simulink library "Library_Muscle_implementation_Ver_01"  (R2020a)
settings: Solver=VariableStepAuto  StartTime=0.0  StopTime=10.0  RelTol=1e-3
undefined symbols (not defined in the file or in its folder): Gait_trajectory_matrix, Param_Mus, X, Y, Z
libraries: sm_lib x8, $bdroot x3, nesl_utility x3, simulink x1, simulink_extras x1
settings Model: Creator=Tobi  LastModifiedBy=Tobi

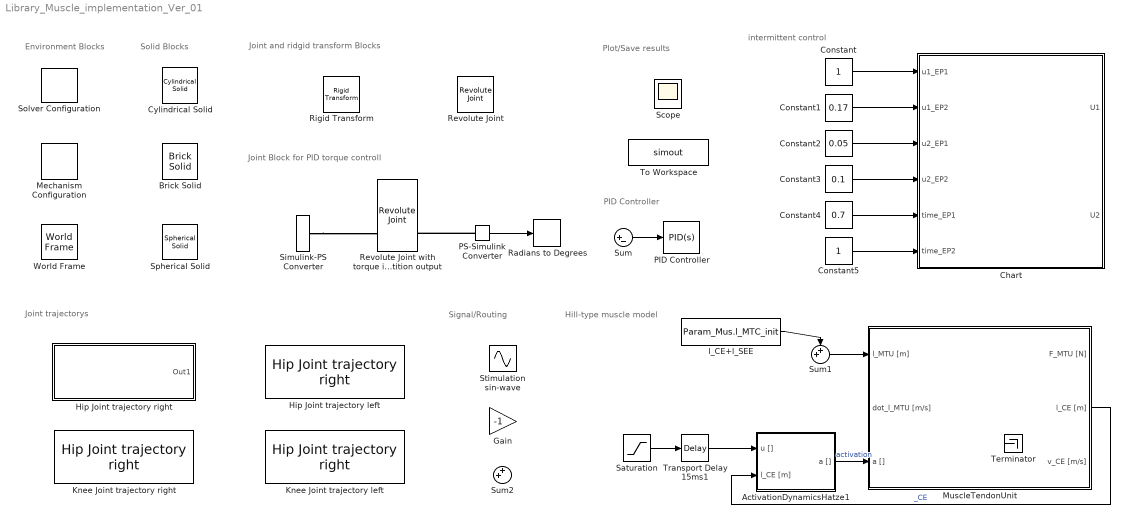
== system Library_Muscle_implementation_Ver_01 ==
  note: Signal/Routing
  note: intermittent control
  note: Joint trajectorys
  note: Plot/Save results
  note: Joint Block for PID torque controll
  note: Solid Blocks
  note: Joint and ridgid transform Blocks
  note: Environment Blocks
  note: PID Controller
  note: Hill-type muscle model
  ActivationDynamicsHatze1 : Subsystem  mask(Activation Dynamics){Act_Param=Param_Mus.ActDyn, Mus_Param=Param_Mus}
      mask prompts: Act_Param "Activation Parameter Struct"; Mus_Param "Muscle Parameter Struct"
      mask help:
      | This block solves the ODE linking neural muscle stimulation u(t) to muscle
      | activity a(t).
      mask Display: %text(.35,.3, 'Aktivierung')
  Brick Solid : sm_lib/Body Elements/Brick Solid  GraphicAmbientColor=[0.15 0.15 0.15 1.0]  BasedOnType=Density  BrickDimensions=[1 1 1]  BrickDimensionUnits=m  CenterOfMass=[0 0 0]  CenterOfMassUnits=m  GraphicDiffuseColor=[0.5 0.5 0.5]  Density=1000  DensityUnits=kg/m^3  DoExposeReferenceFrame=on  GraphicEmissiveColor=[0.0 0.0 0.0 1.0]  ExportEntireGeometry=off  SerializedFrames=<Frames/>  MarkerShape=Sphere  MarkerSize=10  GraphicType=FromGeometry  InertiaType=CalculateFromGeometry  Mass=1  MassUnits=kg  MomentsOfInertia=[1 1 1]  MomentsOfInertiaUnits=kg*m^2  GraphicOpacity=1.0  ProductsOfInertia=[0 0 0]  ProductsOfInertiaUnits=kg*m^2  GraphicShininess=75  GraphicSpecularColor=[0.5 0.5 0.5 1.0]  GraphicVisPropType=SimpleVisualProperties
  Chart : Stateflow chart  TreatAsAtomicUnit=on
  Constant : Constant
  Constant1 : Constant  Value=0.17
  Constant2 : Constant  Value=0.05
  Constant3 : Constant  Value=0.1
  Constant4 : Constant  Value=0.7
  Constant5 : Constant
  Cylindrical Solid : sm_lib/Body Elements/Cylindrical Solid  GraphicAmbientColor=[0.15 0.15 0.15 1.0]  BasedOnType=Density  CenterOfMass=[0 0 0]  CenterOfMassUnits=m  GraphicDiffuseColor=[0.5 0.5 0.5]  CylinderLength=1  CylinderLengthUnits=m  CylinderRadius=1  CylinderRadiusUnits=m  Density=1000  DensityUnits=kg/m^3  DoExposeReferenceFrame=on  GraphicEmissiveColor=[0.0 0.0 0.0 1.0]  ExportEntireGeometry=off  SerializedFrames=<Frames/>  MarkerShape=Sphere  MarkerSize=10  GraphicType=FromGeometry  InertiaType=CalculateFromGeometry  Mass=1  MassUnits=kg  MomentsOfInertia=[1 1 1]  MomentsOfInertiaUnits=kg*m^2  GraphicOpacity=1.0  ProductsOfInertia=[0 0 0]  ProductsOfInertiaUnits=kg*m^2  GraphicShininess=75  GraphicSpecularColor=[0.5 0.5 0.5 1.0]  GraphicVisPropType=SimpleVisualProperties
  Gain : Gain  Gain=-1
  Hip Joint trajectory left : $bdroot/Hip Joint trajectory right   SystemSampleTime=-1  Latency=0  AutoFrameSizeCalculation=off
      link override n-D Lookup Table: Table=Gait_trajectory_matrix(:,2)
  "Hip Joint trajectory right " : Subsystem
  Knee Joint trajectory left : $bdroot/Hip Joint trajectory right   SystemSampleTime=-1  Latency=0  AutoFrameSizeCalculation=off
      link override n-D Lookup Table: Table=Gait_trajectory_matrix(:,4)
  Knee Joint trajectory right : $bdroot/Hip Joint trajectory right   SystemSampleTime=-1  Latency=0  AutoFrameSizeCalculation=off
      link override n-D Lookup Table: Table=Gait_trajectory_matrix(:,5)
  Mechanism Configuration : sm_lib/Utilities/Mechanism Configuration  UniformGravity=Constant  GravityVector=[0 0 -9.80665]  GravityUnits=m/s^2  LinearizationDelta=0.001
  MuscleTendonUnit : Subsystem  mask(Muscle Tendon Complex Model){Mus_Param=Param_Mus}
      mask prompts: Mus_Param "Muscle parameter struct"
      mask help: This block returns the muscle tendon complex (MTC) force based on muscle length l_MTC, contraction velocity dot_l_MTC, and activity q
      mask Help:
      | Copyright (c) 2013, D. Haeufle, M. Guenther, A. Bayer, and S. Schmitt
      | All rights reserved.
      | 
      | Redistribution and use in source and binary forms, with or without modification, are permitted provided that the following conditions are met:
      | 
      |     Redistributions of source code must retain the above copyright notice, this list of conditions and the following disclaimer.
      |     Redistributions in binary form must reproduce the above copyright notice, this list of conditions and the following disclaimer in the documentation and/or other materials provided with the distribution.
      |     Neither the name of the <ORGANIZATION> nor the names of its contributors may be used to endorse or promote products derived from this software without specific prior written permission.
      | 
      | THIS SOFTWARE IS PROVIDED BY THE COPYRIGHT HOLDERS AND CONTRIBUTORS "AS IS" AND ANY EXPRESS OR IMPLIED WARRANTIES, INCLUDING, BUT NOT LIMITED TO, THE IMPLIED WARRANTIES OF MERCHANTABILITY AND FITNESS FOR A PARTICULAR PURPOSE ARE DISCLAIMED. IN NO EVENT SHALL THE COPYRIGHT HOLDER OR CONTRIBUTORS BE LIABLE FOR ANY DIRECT, INDIRECT, INCIDENTAL, SPECIAL, EXEMPLARY, OR CONSEQUENTIAL DAMAGES (INCLUDING, BUT NOT LIMITED TO, PROCUREMENT OF SUBSTITUTE GOODS OR SERVICES; LOSS OF USE, DATA, OR PROFITS; OR BUSINESS INTERRUPTION) HOWEVER CAUSED AND ON ANY THEORY OF LIABILITY, WHETHER IN CONTRACT, STRICT LIABILITY, OR TORT (INCLUDING NEGLIGENCE OR OTHERWISE) ARISING IN ANY WAY OUT OF THE USE OF THIS SOFTWARE, EVEN IF ADVISED OF THE POSSIBILITY OF SUCH DAMAGE.
      mask Display: patch([4 4 4 4 3.5 3 2.6 2.2 2 2.2 2.6 3 3.5 4 4 4 4 7 7 7 7 7.5 8 8.4 8.8 9 8.8 8.4 8 7.5 7 7 7 7 4]/20+0.2, [0 2:17 17:-1:2 0 0]/17,[1 0 0])
  PID Controller : simulink/Continuous/PID Controller  Controller=PID  Form=Parallel  TimeDomain=Continuous-time  UseExternalTs=off  SampleTime=-1  IntegratorMethod=Forward Euler  FilterMethod=Forward Euler  ControllerParametersSource=internal  P=1  I=1  D=0  UseFilter=on  N=100  TunerSelectOption=Transfer Function Based (PID Tuner App)  InitialConditionSource=internal  InitialConditionForIntegrator=0  InitialConditionForFilter=0  DifferentiatorICPrevScaledInput=0  ExternalReset=none  TrackingMode=off  Kt=1  LimitOutput=off  UpperSaturationLimit=inf  LowerSaturationLimit=-inf  LinearizeAsGain=on  AntiWindupMode=none  Kb=1  POutMin=[]  POutMax=[]  IOutMin=[]  IOutMax=[]  DOutMin=[]  DOutMax=[]  NOutMin=[]  NOutMax=[]  SumOutMin=[]  SumOutMax=[]  SaturationOutMin=[]  SaturationOutMax=[]  PParamMin=[]  PParamMax=[]  IParamMin=[]  IParamMax=[]  DParamMin=[]  DParamMax=[]  NParamMin=[]  NParamMax=[]  KbParamMin=[]  KbParamMax=[]  KtParamMin=[]  KtParamMax=[]  KbOutMin=[]  KbOutMax=[]  KtOutMin=[]  KtOutMax=[]  IntegratorOutMin=[]  IntegratorOutMax=[]  FilterOutMin=[]  FilterOutMax=[]  SumI1OutMin=[]  SumI1OutMax=[]  SumI2OutMin=[]  SumI2OutMax=[]  SumI3OutMin=[]  SumI3OutMax=[]  SumI4OutMin=[]  SumI4OutMax=[]  SumDOutMin=[]  SumDOutMax=[]  DifferentiatorOutMin=[]  DifferentiatorOutMax=[]  FilterDiffOutCoefMin=[]  FilterDiffOutCoefMax=[]  ReciprocalOutMin=[]  ReciprocalOutMax=[]  SumDenOutMin=[]  SumDenOutMax=[]  SumNumOutMin=[]  SumNumOutMax=[]  DivideOutMin=[]  DivideOutMax=[]  UdiffTsProdOutMin=[]  UdiffTsProdOutMax=[]  NTsProdOutMin=[]  NTsProdOutMax=[]  UintegralTsProdOutMin=[]  UintegralTsProdOutMax=[]  UngainTsProdOutMin=[]  UngainTsProdOutMax=[]  IntegratorContinuousStateAttributes=''  IntegratorStateMustResolveToSignalObject=off  IntegratorRTWStateStorageClass=Auto  FilterContinuousStateAttributes=''  FilterStateMustResolveToSignalObject=off  FilterRTWStateStorageClass=Auto  ParallelPVariant=InternalParameters  IdealPVariant=Disabled  IVariant=InternalParameters  DVariant=InternalParameters  IntegratorVariant=Continuous  SatVariant=Disabled  AWVariant=Passthrough  PCopyVariant=Disabled  TRVariant=Disabled  FdbkBlocksVariant=Forward  IdealPFdbkVariant=Disabled  SatFdbkVariant=Disabled  DerivativeFilterVariant=ContFilter  NVariant=InternalParameters  NCopyVariant=Disabled  FilterICVariant=InternalICsFilter  IntegratorICVariant=InternalICs  ExternalResetVariant=Disabled  TRSumVariant=Passthrough  SumFdbkVariant=Disabled  SumVariant=Sum_PID  TsampFilterVariant=InternalTs  TsampNgainVariant=Passthrough  TsampIntegralVariant=Passthrough
  PS-Simulink Converter : nesl_utility/PS-Simulink Converter  PhysicalDomain=network_engine_domain  SubClassName=ps_output  LeftPortType=input  RightPortType=output  PseudoPeriodic=off  Frequencies=[]  Unit=1  AffineConversion=off
  Radians to Degrees : simulink_extras/Transformations/Radians to Degrees
  Revolute Joint : sm_lib/Joints/Revolute Joint  JointMode=Normal  SenseConstraintForce=off  SenseConstraintForceX=off  SenseConstraintForceY=off  SenseConstraintForceZ=off  SenseConstraintTorque=off  SenseConstraintTorqueX=off  SenseConstraintTorqueY=off  SenseConstraintTorqueZ=off  SenseTotalForce=off  SenseTotalForceX=off  SenseTotalForceY=off  SenseTotalForceZ=off  SenseTotalTorque=off  SenseTotalTorqueX=off  SenseTotalTorqueY=off  SenseTotalTorqueZ=off  CompositeWrenchDir=FollowerOnBase  CompositeWrenchFrame=BaseFrame  EquilibriumPosition=0  EquilibriumPositionUnits=deg  SpringStiffness=0  SpringStiffnessUnits=N*m/deg  DampingCoefficient=0  DampingCoefficientUnits=N*m/(deg/s)  TorqueActuationMode=NoTorque  MotionActuationMode=ComputedMotion  SensePosition=off  SenseVelocity=off  SenseAcceleration=off  SenseTorqueForce=off  SenseLowerLimitTorqueForce=off  SenseUpperLimitTorqueForce=off  LowerLimitSpecify=off  LowerLimitBound=-90  LowerLimitBoundUnits=deg  LowerLimitStiffness=1e4  LowerLimitStiffnessUnits=N*m/deg  LowerLimitDamping=10  LowerLimitDampingUnits=N*m/(deg/s)  LowerLimitTransitionRegionWidth=0.1  LowerLimitTransitionRegionWidthUnits=deg  UpperLimitSpecify=off  UpperLimitBound=90  UpperLimitBoundUnits=deg  UpperLimitStiffness=1e4  UpperLimitStiffnessUnits=N*m/deg  UpperLimitDamping=10  UpperLimitDampingUnits=N*m/(deg/s)  UpperLimitTransitionRegionWidth=0.1  UpperLimitTransitionRegionWidthUnits=deg  PositionTargetSpecify=off  PositionTargetPriority=High  PositionTargetValue=0  PositionTargetValueUnits=deg  VelocityTargetSpecify=off  VelocityTargetPriority=High  VelocityTargetValue=0  VelocityTargetValueUnits=deg/s
  "Revolute Joint with torque input and postition output " : sm_lib/Joints/Revolute Joint  JointMode=Normal  SenseConstraintForce=off  SenseConstraintForceX=off  SenseConstraintForceY=off  SenseConstraintForceZ=off  SenseConstraintTorque=off  SenseConstraintTorqueX=off  SenseConstraintTorqueY=off  SenseConstraintTorqueZ=off  SenseTotalForce=off  SenseTotalForceX=off  SenseTotalForceY=off  SenseTotalForceZ=off  SenseTotalTorque=off  SenseTotalTorqueX=off  SenseTotalTorqueY=off  SenseTotalTorqueZ=off  CompositeWrenchDir=FollowerOnBase  CompositeWrenchFrame=BaseFrame  EquilibriumPosition=0  EquilibriumPositionUnits=deg  SpringStiffness=0  SpringStiffnessUnits=N*m/deg  DampingCoefficient=0  DampingCoefficientUnits=N*m/(deg/s)  TorqueActuationMode=InputTorque  MotionActuationMode=ComputedMotion  SensePosition=on  SenseVelocity=off  SenseAcceleration=off  SenseTorqueForce=off  SenseLowerLimitTorqueForce=off  SenseUpperLimitTorqueForce=off  LowerLimitSpecify=off  LowerLimitBound=-90  LowerLimitBoundUnits=deg  LowerLimitStiffness=1e4  LowerLimitStiffnessUnits=N*m/deg  LowerLimitDamping=10  LowerLimitDampingUnits=N*m/(deg/s)  LowerLimitTransitionRegionWidth=0.1  LowerLimitTransitionRegionWidthUnits=deg  UpperLimitSpecify=off  UpperLimitBound=90  UpperLimitBoundUnits=deg  UpperLimitStiffness=1e4  UpperLimitStiffnessUnits=N*m/deg  UpperLimitDamping=10  UpperLimitDampingUnits=N*m/(deg/s)  UpperLimitTransitionRegionWidth=0.1  UpperLimitTransitionRegionWidthUnits=deg  PositionTargetSpecify=off  PositionTargetPriority=High  PositionTargetValue=0  PositionTargetValueUnits=deg  VelocityTargetSpecify=off  VelocityTargetPriority=High  VelocityTargetValue=0  VelocityTargetValueUnits=deg/s
  Rigid Transform : sm_lib/Frames and Transforms/Rigid Transform  TranslationMethod=Cartesian  TranslationStandardOffset=0  TranslationLengthUnit=m  TranslationStandardAxis=+Z  TranslationCartesianOffset=[0 0 0]  TranslationROffset=0  TranslationROffsetUnits=m  TranslationZOffset=0  TranslationZOffsetUnits=m  TranslationThetaOffset=0  TranslationThetaOffsetUnits=deg  RotationMethod=StandardAxis  RotationAngleUnits=deg  RotationStandardAxis=+X  RotationAngle=0.0  RotationArbitraryAxis=[0 0 1]  FollAlignAxisA=+X  BaseAlignAxisA=+Y  FollAlignAxisB=+Y  BaseAlignAxisB=+Z  RotationSequenceAxes=FollowerAxes  RotationSequence=XYX  RotationSequenceAngles=[0 0 0]  RotationSequenceAnglesUnits=deg  RotationMatrix=[1 0 0; 0 1 0; 0 0 1]
  Saturation : Saturate  UpperLimit=1  LowerLimit=0.001
  Scope : Scope
  Simulink-PS Converter : nesl_utility/Simulink-PS Converter  PhysicalDomain=network_engine_domain  SubClassName=ps_input  LeftPortType=input  RightPortType=output  PseudoPeriodic=off  Frequencies=[]  NoiseDistribution=none  NoiseParameters=[]  Unit=1  AffineConversion=off  FilteringAndDerivatives=zero  SimscapeFilterOrder=2  InputFilterTimeConstant=0.001  UdotUserProvided=0
  Solver Configuration : nesl_utility/Solver Configuration  PhysicalDomain=network_engine_domain  SubClassName=solver  LeftPortType=input  RightPortType=generic  Tones=[]  Harmonics=[]  SimulateNoise=off  Profile=off  UseLocalSampling=off  EnableSwitchedLinearOptims=on  FrequencyDomain=off  UseCCode=off  RelTol=0.001  AbsTol=1e-06  MinStep=1e-09  ToWorkspace=off  RevertToSquareIcSolve=off  NumHomotopyIterations=100  PhasorMode=off  PhasorModeNumHarmonics=1  DoDC=off  ResidualTolerance=1e-09  UseLocalSolver=off  LocalSolverChoice=NE_BACKWARD_EULER_ADVANCER  LocalSolverSampleTime=0.001  DoFixedCost=off  MaxNonlinIter=3  MaxModeIter=2  LinearAlgebra=auto  EquationFormulation=NE_TIME_EF  DelaysMemoryBudget=1024  AutomaticFiltering=on  FilteringTimeConstant=0.001  PartitionStorageMethod=AS_NEEDED  PartitionMemoryBudget=1024  PartitionMethod=ROBUST
  Spherical Solid : sm_lib/Body Elements/Spherical Solid  GraphicAmbientColor=[0.15 0.15 0.15 1.0]  BasedOnType=Density  CenterOfMass=[0 0 0]  CenterOfMassUnits=m  GraphicDiffuseColor=[0.0 0.0 0.0]  Density=1000  DensityUnits=kg/m^3  DoExposeReferenceFrame=on  GraphicEmissiveColor=[0.0 0.0 0.0 1.0]  ExportEntireGeometry=off  SerializedExposedGeometries=<ExposedGeometries/>  SerializedFrames=<Frames/>  MarkerShape=Sphere  MarkerSize=10  GraphicType=FromGeometry  InertiaType=PointMass  Mass=0  MassUnits=kg  MomentsOfInertia=[1 1 1]  MomentsOfInertiaUnits=kg*m^2  GraphicOpacity=1.0  ProductsOfInertia=[0 0 0]  ProductsOfInertiaUnits=kg*m^2  GraphicShininess=75  GraphicSpecularColor=[0.5 0.5 0.5 1.0]  SphereRadius=Joint_radius  SphereRadiusUnits=m  GraphicVisPropType=SimpleVisualProperties
  Stimulation sin-wave : Sin  Amplitude=0.25  Bias=0.45  Frequency=3  Phase=-pi/2  SampleTime=0
  Sum : Sum  Inputs=|+-
  Sum1 : Sum  Inputs=++|
  Sum2 : Sum  Inputs=++|
  Terminator : Terminator
  To Workspace : ToWorkspace  VariableName=simout  SaveFormat=Structure With Time  SampleTime=-1
  Transport Delay 15ms1 : TransportDelay  DelayTime=0.015  InitialOutput=Param_Mus.ActDyn.u_init
  World Frame : sm_lib/Frames and Transforms/World Frame
  l_CE+l_SEE : Constant  Value=Param_Mus.l_MTC_init
  wires:
  PS-Simulink Converter/1 -> Radians to Degrees/1
  Sum/1 -> PID Controller/1
  l_CE+l_SEE/1 -> Sum1/1
  MuscleTendonUnit/2(l_CE [m]) -> ActivationDynamicsHatze1/2(l_CE [m])  "_CE"
  Transport Delay 15ms1/1 -> ActivationDynamicsHatze1/1(u [])
  ActivationDynamicsHatze1/1(a []) -> MuscleTendonUnit/3(a [])  "activation"
  ? -> Terminator/1  "v_CE"
  Sum1/1 -> MuscleTendonUnit/1(l_MTU [m])
  Constant2/1 -> Chart/3(u2_EP1)
  Constant3/1 -> Chart/4(u2_EP2)
  Constant/1 -> Chart/1(u1_EP1)
  Constant1/1 -> Chart/2(u1_EP2)
  Constant4/1 -> Chart/5(time_EP1)
  Constant5/1 -> Chart/6(time_EP2)
  Saturation/1 -> Transport Delay 15ms1/1
  connections:
  PS-Simulink Converter/LConn1 -- "Revolute Joint with torque input and postition output "/RConn2
  Simulink-PS Converter/RConn1 -- "Revolute Joint with torque input and postition output "/LConn2

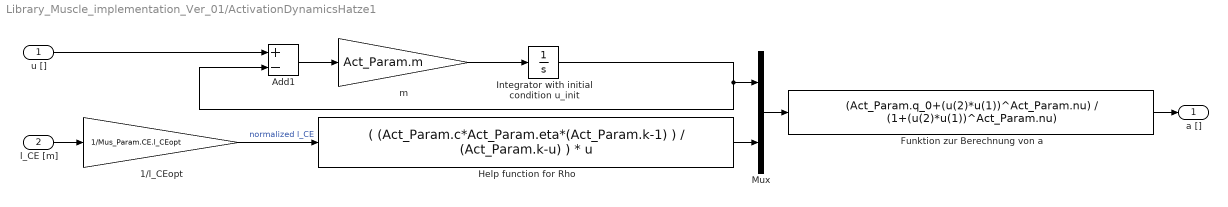
== system Library_Muscle_implementation_Ver_01/ActivationDynamicsHatze1 ==
  u [] : Inport
  l_CE [m] : Inport  Port=2
  1/l_CEopt : Gain  Gain=1/Mus_Param.CE.l_CEopt
  Add1 : Sum  Inputs=+-
  Funktion zur Berechnung von a : Fcn  Expr=(Act_Param.q_0+(u(2)*u(1))^Act_Param.nu) / (1+(u(2)*u(1))^Act_Param.nu)
  Help function for Rho : Fcn  Expr=( (Act_Param.c*Act_Param.eta*(Act_Param.k-1) ) / (Act_Param.k-u) ) * u
  Integrator with initial condition u_init : Integrator  InitialCondition=Act_Param.u_init
  Mux : Mux  Inputs=2
  m : Gain  Gain=Act_Param.m
  a [] : Outport  VectorParamsAs1DForOutWhenUnconnected=off
  wires:
  Add1/1 -> m/1
  m/1 -> Integrator with initial condition u_init/1
  Integrator with initial condition u_init/1 -> Add1/2, Mux/1
  Help function for Rho/1 -> Mux/2
  Mux/1 -> Funktion zur Berechnung von a/1
  l_CE [m]/1 -> 1/l_CEopt/1
  Funktion zur Berechnung von a/1 -> a []/1
  u []/1 -> Add1/1
  1/l_CEopt/1 -> Help function for Rho/1  "normalized l_CE"

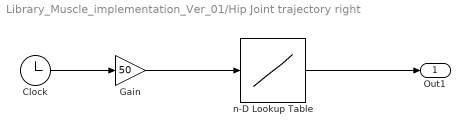
== system Library_Muscle_implementation_Ver_01/Hip Joint trajectory right  ==
  Clock : Clock
  Gain : Gain  Gain=50
  n-D Lookup Table : Lookup_n-D  NumberOfTableDimensions=1  BreakpointsSpecification=Even spacing  BreakpointsForDimension3=[5, 7]  Table=Gait_trajectory_matrix(:,3)  InternalRulePriority=Speed  RndMeth=Simplest  InputSameDT=on
  Out1 : Outport
  wires:
  n-D Lookup Table/1 -> Out1/1
  Clock/1 -> Gain/1
  Gain/1 -> n-D Lookup Table/1

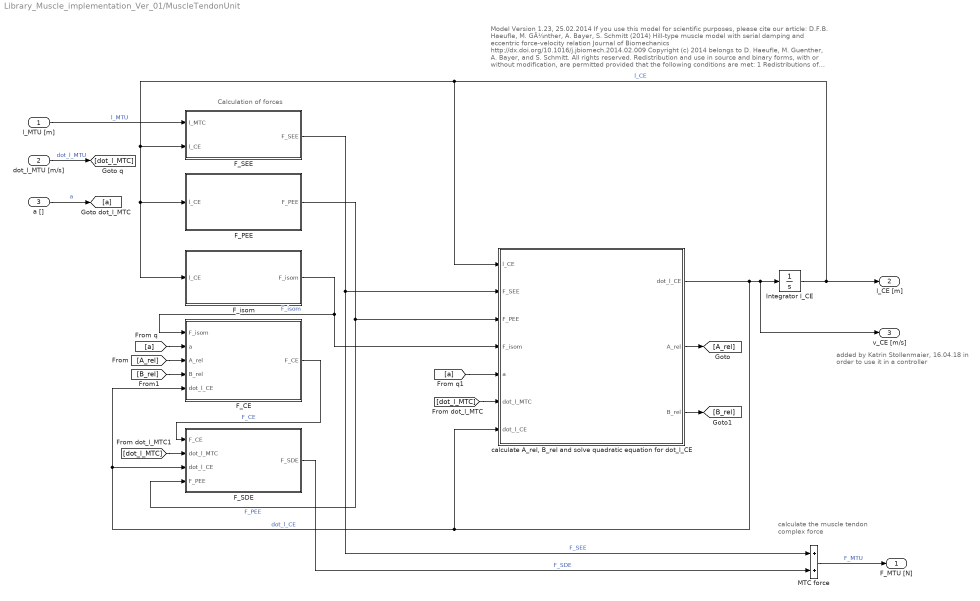
== system Library_Muscle_implementation_Ver_01/MuscleTendonUnit ==
  note: added by Katrin Stollenmaier,
      | 16.04.18 in order to use it in a controller
  note: Calculation of forces
  note: calculate the
      | muscle tendon complex
      | force
  note: Model Version 1.23, 25.02.2014
      |
      | If you use this model for scientific purposes, please cite our article:
      | D.F.B. Haeufle, M. GÃ¼nther, A. Bayer, S. Schmitt (2014)
      | Hill-type muscle model with serial damping and eccentric force-velocity relation
      | Journal of Biomechanics http://dx.doi.org/10.1016/j.jbiomech.2014.02.009
      |
      |
      | Copyright (c) 2014 belongs to D. Haeufle, M. Guenther, A. Bayer, and S. Schmitt. All rights reserved.
      | Redistribution and use in source and binary forms, with or without modification, are permitted provided that the following conditions are met:
      |
      |  1 Redistributions of source code must retain the above copyright notice,
      |    this list of conditions and the following disclaimer.
      |  2 Redistributions in binary form must reproduce the above copyright
      |    notice, this list of conditions and the following disclaimer in the
      |    documentation and/or other materials provided with the distribution.
      |  3 Neither the name of the owner nor the names of its contributors may be
      |    used to endorse or promote products derived from this software without
      |    specific prior written permission.
      |
      | THIS SOFTWARE IS PROVIDED BY THE COPYRIGHT HOLDERS AND CONTRIBUTORS "AS IS"
      | AND ANY EXPRESS OR IMPLIED WARRANTIES, INCLUDING, BUT NOT LIMITED TO, THE IMPLIED WARRANTIES OF
      | MERCHANTABILITY AND FITNESS FOR A PARTICULAR PURPOSE ARE DISCLAIMED.
      |  IN NO EVENT SHALL THE COPYRIGHT HOLDER BE LIABLE FOR ANY DIRECT, INDIRECT,
      | INCIDENTAL, SPECIAL, EXEMPLARY, OR CONSEQUENTIAL DAMAGES (INCLUDING, BUT
      | NOT LIMITED TO, PROCUREMENT OF SUBSTITUTE GOODS OR SERVICES; LOSS
      | OF USE, DATA, OR PROFITS; OR BUSINESS INTERRUPTION) HOWEVER CAUSED AND ON ANY
      | THEORY OF LIABILITY, WHETHER IN CONTRACT, STRICT LIABILITY, OR TORT (INCLUDING
      | NEGLIGENCE OR OTHERWISE) ARISING IN ANY WAY OUT OF THE USE OF THIS SOFTWARE,
      | EVEN IF ADVISED OF THE POSSIBILITY OF SUCH DAMAGE.
  l_MTU [m] : Inport
  dot_l_MTU [m/s] : Inport  Port=2
  a [] : Inport  Port=3
  F_CE : Subsystem
  F_PEE : Subsystem
  F_SDE : Subsystem
  F_SEE : Subsystem
  F_isom : Subsystem
  Integrator l_CE : Integrator  InitialCondition=Mus_Param.CE.l_CE_init
  MTC force : Sum
  "calculate A_rel, B_rel and solve quadratic equation for dot_l_CE" : Subsystem
  F_MTU [N] : Outport  VectorParamsAs1DForOutWhenUnconnected=off
  l_CE [m] : Outport  Port=2  VectorParamsAs1DForOutWhenUnconnected=off
  "v_CE [m/s] " : Outport  Port=3  VectorParamsAs1DForOutWhenUnconnected=off
  wires:
  F_isom/1(F_isom) -> "calculate A_rel, B_rel and solve quadratic equation for dot_l_CE"/4(F_isom), F_CE/1(F_isom)  "F_isom"
  F_PEE/1(F_PEE) -> F_SDE/4(F_PEE), "calculate A_rel, B_rel and solve quadratic equation for dot_l_CE"/3(F_PEE)  "F_PEE"
  F_SEE/1(F_SEE) -> MTC force/1, "calculate A_rel, B_rel and solve quadratic equation for dot_l_CE"/2(F_SEE)  "F_SEE"
  Integrator l_CE/1 -> l_CE [m]/1, "calculate A_rel, B_rel and solve quadratic equation for dot_l_CE"/1(l_CE), F_SEE/2(l_CE), F_isom/1(l_CE), F_PEE/1(l_CE)  "l_CE"
  F_CE/1(F_CE) -> F_SDE/1(F_CE)  "F_CE"
  F_SDE/1(F_SDE) -> MTC force/2  "F_SDE"
  MTC force/1 -> F_MTU [N]/1  "F_MTU"
  l_MTU [m]/1 -> F_SEE/1(l_MTC)  "l_MTU"
  "calculate A_rel, B_rel and solve quadratic equation for dot_l_CE"/1("dot_l_CE ") -> "calculate A_rel, B_rel and solve quadratic equation for dot_l_CE"/7(dot_l_CE), F_CE/5(dot_l_CE), F_SDE/3(dot_l_CE), "v_CE [m/s] "/1, Integrator l_CE/1  "dot_l_CE"
  [a] -> F_CE/2(a)
  [a] -> "calculate A_rel, B_rel and solve quadratic equation for dot_l_CE"/5("a ")
  [dot_l_MTC] -> "calculate A_rel, B_rel and solve quadratic equation for dot_l_CE"/6(dot_l_MTC)
  [dot_l_MTC] -> F_SDE/2(dot_l_MTC)
  "calculate A_rel, B_rel and solve quadratic equation for dot_l_CE"/2(A_rel) -> [A_rel]
  "calculate A_rel, B_rel and solve quadratic equation for dot_l_CE"/3(B_rel) -> [B_rel]
  [A_rel] -> F_CE/3(A_rel)
  [B_rel] -> F_CE/4(B_rel)
  dot_l_MTU [m/s]/1 -> [dot_l_MTC]  "dot_l_MTU"
  a []/1 -> [a]  "a"

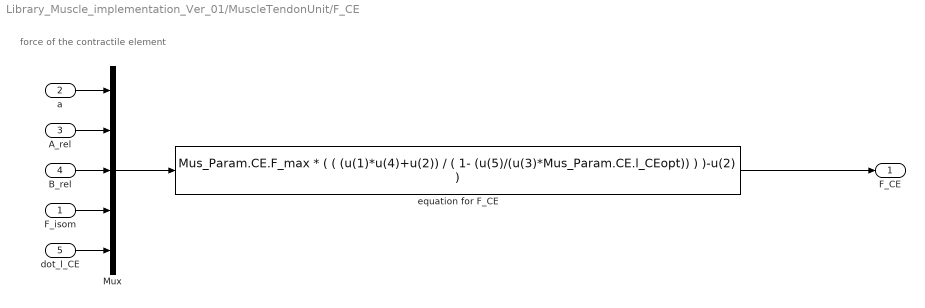
== system Library_Muscle_implementation_Ver_01/MuscleTendonUnit/F_CE ==
  note: force of the contractile element
  F_isom : Inport
  a : Inport  Port=2
  A_rel : Inport  Port=3
  B_rel : Inport  Port=4
  dot_l_CE : Inport  Port=5
  Mux : Mux  Inputs=5
  equation for F_CE : Fcn  Expr="Mus_Param.CE.F_max * (  ( (u(1)*u(4)+u(2)) / ( 1- (u(5)/(u(3)*Mus_Param.CE.l_CEopt)) ) )-u(2) )"
  F_CE : Outport  VectorParamsAs1DForOutWhenUnconnected=off
  wires:
  Mux/1 -> equation for F_CE/1
  a/1 -> Mux/1
  A_rel/1 -> Mux/2
  B_rel/1 -> Mux/3
  F_isom/1 -> Mux/4
  dot_l_CE/1 -> Mux/5
  equation for F_CE/1 -> F_CE/1

== system Library_Muscle_implementation_Ver_01/MuscleTendonUnit/F_PEE ==
  note: Parallel elastic element force
      |
      | is only calculated if l_CE>PEE slack length
      | to avoid complex numbers with
      | non-integer exponents
  l_CE : Inport
  "F_PEE " : Subsystem
  l_PEE > slack length? : Fcn  Expr=(u>=Mus_Param.PEE.l_PEE0)
  F_PEE : Outport  VectorParamsAs1DForOutWhenUnconnected=off
  wires:
  l_CE/1 -> l_PEE > slack length?/1, "F_PEE "/1(l_PEE)
  "F_PEE "/1(Out1) -> F_PEE/1
  l_PEE > slack length?/1 -> "F_PEE "/Enable

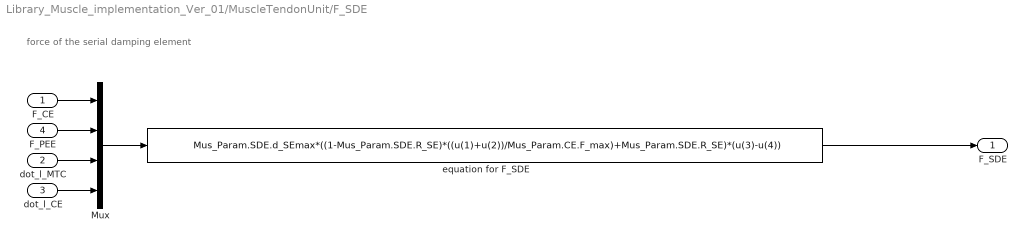
== system Library_Muscle_implementation_Ver_01/MuscleTendonUnit/F_SDE ==
  note: force of the serial damping element
  F_CE : Inport
  dot_l_MTC : Inport  Port=2
  dot_l_CE : Inport  Port=3
  F_PEE : Inport  Port=4
  Mux : Mux
  equation for F_SDE : Fcn  Expr=Mus_Param.SDE.d_SEmax*((1-Mus_Param.SDE.R_SE)*((u(1)+u(2))/Mus_Param.CE.F_max)+Mus_Param.SDE.R_SE)*(u(3)-u(4))
  F_SDE : Outport  VectorParamsAs1DForOutWhenUnconnected=off
  wires:
  Mux/1 -> equation for F_SDE/1
  F_PEE/1 -> Mux/2
  F_CE/1 -> Mux/1
  equation for F_SDE/1 -> F_SDE/1
  dot_l_MTC/1 -> Mux/3
  dot_l_CE/1 -> Mux/4

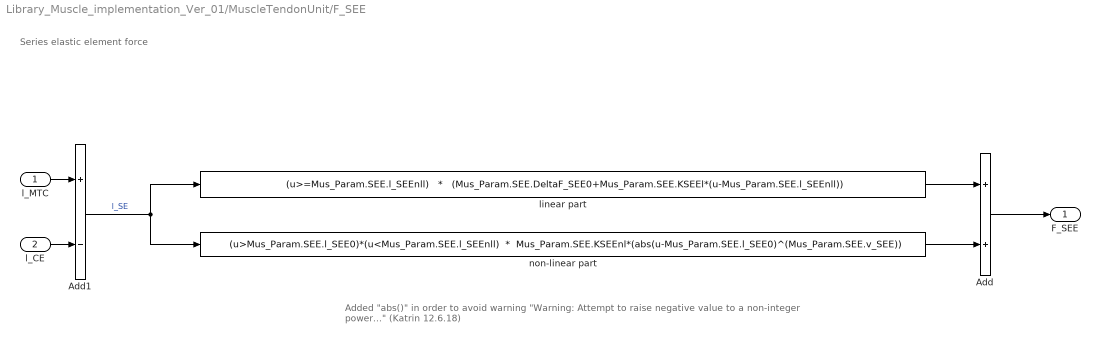
== system Library_Muscle_implementation_Ver_01/MuscleTendonUnit/F_SEE ==
  note: Added "abs()" in order to avoid warning "Warning: Attempt to raise negative value to a non-integer power..."
      | (Katrin 12.6.18)
  note: Series elastic element force
  l_MTC : Inport
  l_CE : Inport  Port=2
  Add : Sum
  Add1 : Sum  Inputs=+-
  linear part : Fcn  Expr="(u>=Mus_Param.SEE.l_SEEnll)   *   (Mus_Param.SEE.DeltaF_SEE0+Mus_Param.SEE.KSEEl*(u-Mus_Param.SEE.l_SEEnll))"
  non-linear part : Fcn  Expr="(u>Mus_Param.SEE.l_SEE0)*(u<Mus_Param.SEE.l_SEEnll)  *  Mus_Param.SEE.KSEEnl*(abs(u-Mus_Param.SEE.l_SEE0)^(Mus_Param.SEE.v_SEE))"
  F_SEE : Outport  VectorParamsAs1DForOutWhenUnconnected=off
  wires:
  linear part/1 -> Add/1
  Add1/1 -> linear part/1, non-linear part/1  "l_SE"
  l_MTC/1 -> Add1/1
  Add/1 -> F_SEE/1
  l_CE/1 -> Add1/2
  non-linear part/1 -> Add/2

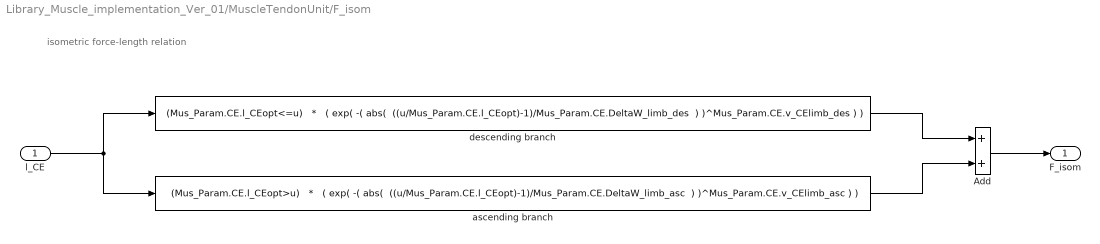
== system Library_Muscle_implementation_Ver_01/MuscleTendonUnit/F_isom ==
  note: isometric force-length relation
  l_CE : Inport
  Add : Sum
  ascending branch : Fcn  Expr="(Mus_Param.CE.l_CEopt>u)   *   ( exp( -( abs(  ((u/Mus_Param.CE.l_CEopt)-1)/Mus_Param.CE.DeltaW_limb_asc  ) )^Mus_Param.CE.v_CElimb_asc ) )"
  descending branch : Fcn  Expr="(Mus_Param.CE.l_CEopt<=u)   *   ( exp( -( abs(  ((u/Mus_Param.CE.l_CEopt)-1)/Mus_Param.CE.DeltaW_limb_des  ) )^Mus_Param.CE.v_CElimb_des ) )"
  F_isom : Outport  VectorParamsAs1DForOutWhenUnconnected=off
  wires:
  descending branch/1 -> Add/1
  ascending branch/1 -> Add/2
  Add/1 -> F_isom/1
  l_CE/1 -> descending branch/1, ascending branch/1

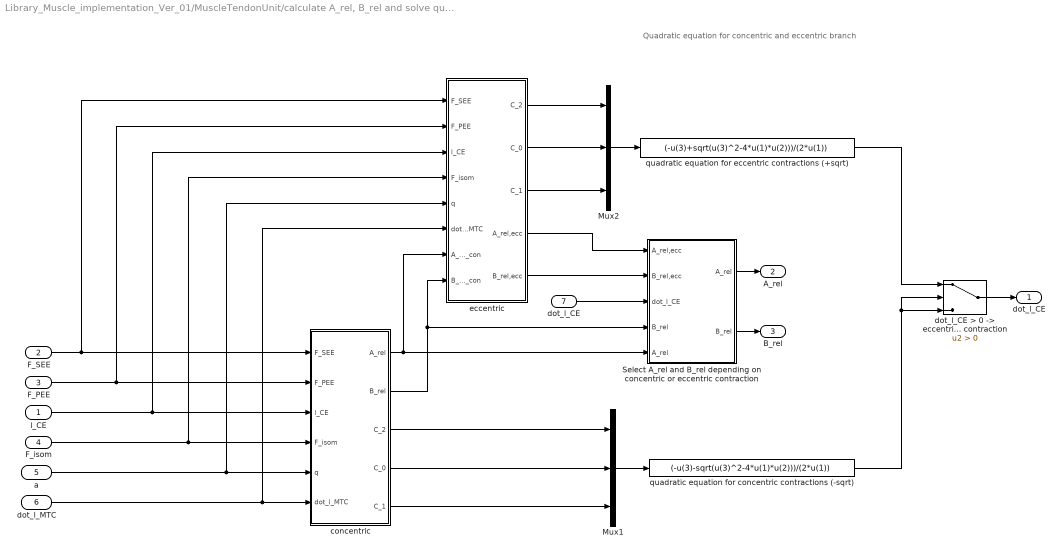
== system Library_Muscle_implementation_Ver_01/MuscleTendonUnit/calculate A_rel, B_rel and solve quadratic equation for dot_l_CE ==
  note: Quadratic equation for concentric and eccentric branch
  l_CE : Inport
  F_SEE : Inport  Port=2
  F_PEE : Inport  Port=3
  F_isom : Inport  Port=4
  "a " : Inport  Port=5
  dot_l_MTC : Inport  Port=6
  dot_l_CE : Inport  Port=7
  Mux1 : Mux  Inputs=3
  Mux2 : Mux  Inputs=3
  Select A_rel and B_rel depending on concentric or eccentric contraction : Subsystem
  concentric : Subsystem
  "dot_l_CE > 0 -> eccentric contraction" : Switch  Criteria=u2 > Threshold  ZeroCross=off
  eccentric : Subsystem
  quadratic equation for concentric contractions (-sqrt) : Fcn  Expr=(-u(3)-sqrt(u(3)^2-4*u(1)*u(2)))/(2*u(1))
  quadratic equation for eccentric contractions (+sqrt) : Fcn  Expr=(-u(3)+sqrt(u(3)^2-4*u(1)*u(2)))/(2*u(1))
  "dot_l_CE " : Outport  VectorParamsAs1DForOutWhenUnconnected=off
  A_rel : Outport  Port=2  VectorParamsAs1DForOutWhenUnconnected=off
  B_rel : Outport  Port=3  VectorParamsAs1DForOutWhenUnconnected=off
  wires:
  dot_l_MTC/1 -> eccentric/6(dot_l_MTC), concentric/6(dot_l_MTC)
  F_PEE/1 -> eccentric/2(F_PEE), concentric/2(F_PEE)
  l_CE/1 -> eccentric/3(l_CE), concentric/3(l_CE)
  concentric/2(B_rel) -> eccentric/8(B_rel_con), Select A_rel and B_rel depending on concentric or eccentric contraction/4(B_rel)
  F_SEE/1 -> eccentric/1(F_SEE), concentric/1(F_SEE)
  F_isom/1 -> eccentric/4(F_isom), concentric/4(F_isom)
  "a "/1 -> eccentric/5(q), concentric/5(q)
  concentric/1(A_rel) -> eccentric/7(A_rel_con), Select A_rel and B_rel depending on concentric or eccentric contraction/5(A_rel)
  "dot_l_CE > 0 -> eccentric contraction"/1 -> "dot_l_CE "/1
  concentric/3("C_2 ") -> Mux1/1
  concentric/4("C_0 ") -> Mux1/2
  concentric/5("C_1 ") -> Mux1/3
  Mux1/1 -> quadratic equation for concentric contractions (-sqrt)/1
  quadratic equation for concentric contractions (-sqrt)/1 -> "dot_l_CE > 0 -> eccentric contraction"/2, "dot_l_CE > 0 -> eccentric contraction"/3
  quadratic equation for eccentric contractions (+sqrt)/1 -> "dot_l_CE > 0 -> eccentric contraction"/1
  Mux2/1 -> quadratic equation for eccentric contractions (+sqrt)/1
  eccentric/1(C_2) -> Mux2/1
  eccentric/2(C_0) -> Mux2/2
  eccentric/3(C_1) -> Mux2/3
  eccentric/4(A_rel,ecc) -> Select A_rel and B_rel depending on concentric or eccentric contraction/1(A_rel,ecc)
  eccentric/5(B_rel,ecc) -> Select A_rel and B_rel depending on concentric or eccentric contraction/2(B_rel,ecc)
  dot_l_CE/1 -> Select A_rel and B_rel depending on concentric or eccentric contraction/3(dot_l_CE)
  Select A_rel and B_rel depending on concentric or eccentric contraction/1(" A_rel") -> A_rel/1
  Select A_rel and B_rel depending on concentric or eccentric contraction/2("B_rel ") -> B_rel/1

== system Library_Muscle_implementation_Ver_01/MuscleTendonUnit/F_PEE/F_PEE  ==
  note: Added "abs()" in order to avoid warning "Warning: Attempt to raise negative value to a non-integer power..."
      | (Katrin 12.6.18)
  l_PEE : Inport
  Enable : EnablePort  StatesWhenEnabling=reset
  "F_PEE " : Fcn  Expr=Mus_Param.PEE.K_PEE*abs(u-Mus_Param.PEE.l_PEE0)^(Mus_Param.PEE.v_PEE)
  Out1 : Outport  InitialOutput=0  VectorParamsAs1DForOutWhenUnconnected=off
  wires:
  l_PEE/1 -> "F_PEE "/1
  "F_PEE "/1 -> Out1/1

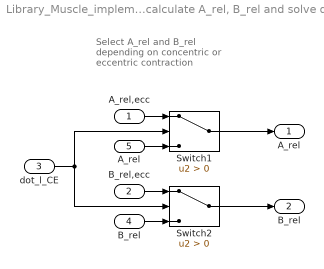
== system Library_Muscle_implementation_Ver_01/MuscleTendonUnit/calculate A_rel, B_rel and solve quadratic equation for dot_l_CE/Select A_rel and B_rel depending on concentric or eccentric contraction ==
  note: Select A_rel and B_rel
      | depending on concentric or
      | eccentric contraction
  A_rel,ecc : Inport
  B_rel,ecc : Inport  Port=2
  dot_l_CE : Inport  Port=3
  B_rel : Inport  Port=4
  A_rel : Inport  Port=5
  Switch1 : Switch  Criteria=u2 > Threshold  ZeroCross=off
  Switch2 : Switch  Criteria=u2 > Threshold  ZeroCross=off
  " A_rel" : Outport  VectorParamsAs1DForOutWhenUnconnected=off
  "B_rel " : Outport  Port=2  VectorParamsAs1DForOutWhenUnconnected=off
  wires:
  dot_l_CE/1 -> Switch1/2, Switch2/2
  Switch1/1 -> " A_rel"/1
  Switch2/1 -> "B_rel "/1
  A_rel,ecc/1 -> Switch1/1
  B_rel,ecc/1 -> Switch2/1
  A_rel/1 -> Switch1/3
  B_rel/1 -> Switch2/3

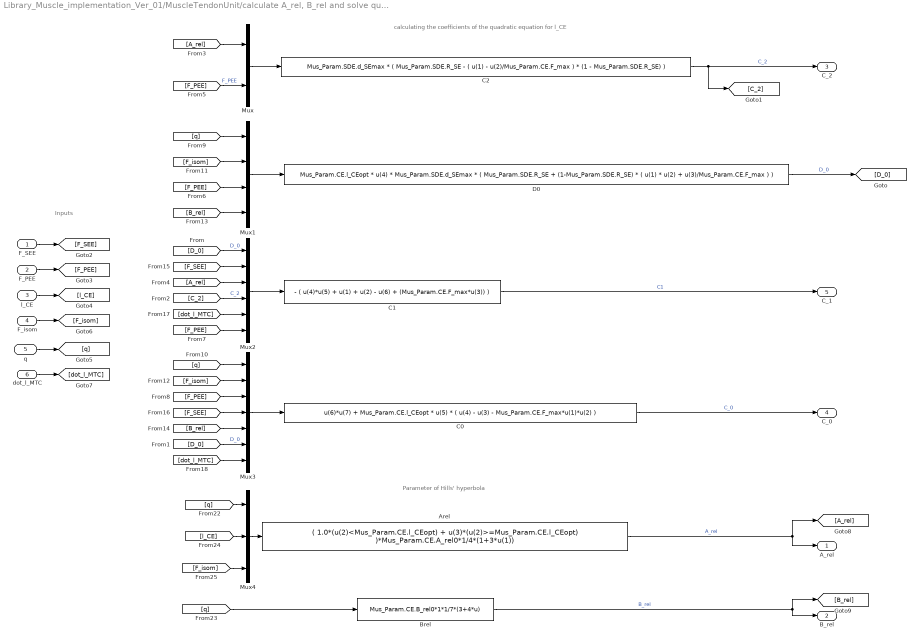
== system Library_Muscle_implementation_Ver_01/MuscleTendonUnit/calculate A_rel, B_rel and solve quadratic equation for dot_l_CE/concentric ==
  note: Inputs
  note: calculating the coefficients of the quadratic equation for l_CE
  note: Parameter of Hills' hyperbola
  F_SEE : Inport
  F_PEE : Inport  Port=2
  l_CE : Inport  Port=3
  F_isom : Inport  Port=4
  q : Inport  Port=5
  dot_l_MTC : Inport  Port=6
  Arel : Fcn  Expr=( 1.0*(u(2)<Mus_Param.CE.l_CEopt) + u(3)*(u(2)>=Mus_Param.CE.l_CEopt) )*Mus_Param.CE.A_rel0*1/4*(1+3*u(1))
  Brel : Fcn  Expr=Mus_Param.CE.B_rel0*1*1/7*(3+4*u)
  C0 : Fcn  Expr=u(6)*u(7) + Mus_Param.CE.l_CEopt * u(5) * ( u(4) - u(3) - Mus_Param.CE.F_max*u(1)*u(2) )
  C1 : Fcn  Expr=- ( u(4)*u(5) + u(1) + u(2) - u(6) + (Mus_Param.CE.F_max*u(3)) )
  C2 : Fcn  Expr=Mus_Param.SDE.d_SEmax * ( Mus_Param.SDE.R_SE - ( u(1) - u(2)/Mus_Param.CE.F_max ) * (1 - Mus_Param.SDE.R_SE) )
  "D0 " : Fcn  Expr=Mus_Param.CE.l_CEopt * u(4) * Mus_Param.SDE.d_SEmax * ( Mus_Param.SDE.R_SE + (1-Mus_Param.SDE.R_SE) * ( u(1) * u(2) + u(3)/Mus_Param.CE.F_max ) )
  Mux : Mux  Inputs=2
  Mux1 : Mux
  Mux2 : Mux  Inputs=6
  Mux3 : Mux  Inputs=7
  Mux4 : Mux  Inputs=3
  A_rel : Outport  VectorParamsAs1DForOutWhenUnconnected=off
  B_rel : Outport  Port=2  VectorParamsAs1DForOutWhenUnconnected=off
  "C_2 " : Outport  Port=3  VectorParamsAs1DForOutWhenUnconnected=off
  "C_0 " : Outport  Port=4  VectorParamsAs1DForOutWhenUnconnected=off
  "C_1 " : Outport  Port=5  VectorParamsAs1DForOutWhenUnconnected=off
  wires:
  Arel/1 -> A_rel/1, [A_rel]  "A_rel"
  dot_l_MTC/1 -> [dot_l_MTC]
  Brel/1 -> [B_rel], B_rel/1  "B_rel"
  Mux/1 -> C2/1
  C2/1 -> "C_2 "/1, [C_2]  "C_2"
  Mux1/1 -> "D0 "/1
  "D0 "/1 -> [D_0]  "D_0"
  Mux2/1 -> C1/1
  [D_0] -> Mux2/1  "D_0"
  [C_2] -> Mux2/4  "C_2"
  C1/1 -> "C_1 "/1  "C1"
  Mux3/1 -> C0/1
  [D_0] -> Mux3/6  "D_0"
  C0/1 -> "C_0 "/1  "C_0"
  [A_rel] -> Mux/1
  F_SEE/1 -> [F_SEE]
  F_PEE/1 -> [F_PEE]
  l_CE/1 -> [l_CE]
  q/1 -> [q]
  F_isom/1 -> [F_isom]
  [A_rel] -> Mux2/3
  [dot_l_MTC] -> Mux3/7
  [F_PEE] -> Mux/2  "F_PEE"
  [q] -> Mux1/1
  [F_isom] -> Mux1/2
  [F_PEE] -> Mux1/3
  [B_rel] -> Mux1/4
  [F_SEE] -> Mux2/2
  [dot_l_MTC] -> Mux2/5
  [F_PEE] -> Mux2/6
  [q] -> Mux3/1
  [F_isom] -> Mux3/2
  [F_PEE] -> Mux3/3
  [F_SEE] -> Mux3/4
  [B_rel] -> Mux3/5
  Mux4/1 -> Arel/1
  [F_isom] -> Mux4/3
  [l_CE] -> Mux4/2
  [q] -> Mux4/1
  [q] -> Brel/1

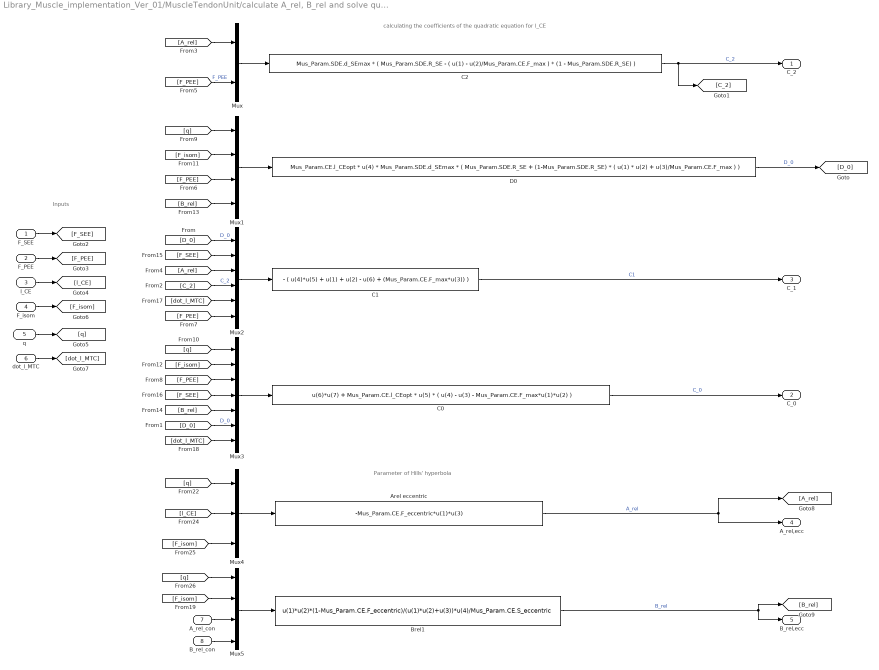
== system Library_Muscle_implementation_Ver_01/MuscleTendonUnit/calculate A_rel, B_rel and solve quadratic equation for dot_l_CE/eccentric ==
  note: Inputs
  note: calculating the coefficients of the quadratic equation for l_CE
  note: Parameter of Hills' hyperbola
  F_SEE : Inport
  F_PEE : Inport  Port=2
  l_CE : Inport  Port=3
  F_isom : Inport  Port=4
  q : Inport  Port=5
  dot_l_MTC : Inport  Port=6
  A_rel_con : Inport  Port=7
  B_rel_con : Inport  Port=8
  Arel eccentric : Fcn  Expr=-Mus_Param.CE.F_eccentric*u(1)*u(3)
  Brel1 : Fcn  Expr=u(1)*u(2)*(1-Mus_Param.CE.F_eccentric)/(u(1)*u(2)+u(3))*u(4)/Mus_Param.CE.S_eccentric
  C0 : Fcn  Expr=u(6)*u(7) + Mus_Param.CE.l_CEopt * u(5) * ( u(4) - u(3) - Mus_Param.CE.F_max*u(1)*u(2) )
  C1 : Fcn  Expr=- ( u(4)*u(5) + u(1) + u(2) - u(6) + (Mus_Param.CE.F_max*u(3)) )
  C2 : Fcn  Expr=Mus_Param.SDE.d_SEmax * ( Mus_Param.SDE.R_SE - ( u(1) - u(2)/Mus_Param.CE.F_max ) * (1 - Mus_Param.SDE.R_SE) )
  "D0 " : Fcn  Expr=Mus_Param.CE.l_CEopt * u(4) * Mus_Param.SDE.d_SEmax * ( Mus_Param.SDE.R_SE + (1-Mus_Param.SDE.R_SE) * ( u(1) * u(2) + u(3)/Mus_Param.CE.F_max ) )
  Mux : Mux  Inputs=2
  Mux1 : Mux
  Mux2 : Mux  Inputs=6
  Mux3 : Mux  Inputs=7
  Mux4 : Mux  Inputs=3
  Mux5 : Mux
  C_2 : Outport  VectorParamsAs1DForOutWhenUnconnected=off
  C_0 : Outport  Port=2  VectorParamsAs1DForOutWhenUnconnected=off
  C_1 : Outport  Port=3  VectorParamsAs1DForOutWhenUnconnected=off
  A_rel,ecc : Outport  Port=4  VectorParamsAs1DForOutWhenUnconnected=off
  B_rel,ecc : Outport  Port=5  VectorParamsAs1DForOutWhenUnconnected=off
  wires:
  Arel eccentric/1 -> A_rel,ecc/1, [A_rel]  "A_rel"
  dot_l_MTC/1 -> [dot_l_MTC]
  Brel1/1 -> [B_rel], B_rel,ecc/1  "B_rel"
  Mux/1 -> C2/1
  C2/1 -> C_2/1, [C_2]  "C_2"
  Mux1/1 -> "D0 "/1
  "D0 "/1 -> [D_0]  "D_0"
  Mux2/1 -> C1/1
  [D_0] -> Mux2/1  "D_0"
  [C_2] -> Mux2/4  "C_2"
  C1/1 -> C_1/1  "C1"
  Mux3/1 -> C0/1
  [D_0] -> Mux3/6  "D_0"
  C0/1 -> C_0/1  "C_0"
  [A_rel] -> Mux/1
  F_SEE/1 -> [F_SEE]
  F_PEE/1 -> [F_PEE]
  l_CE/1 -> [l_CE]
  q/1 -> [q]
  F_isom/1 -> [F_isom]
  [A_rel] -> Mux2/3
  [dot_l_MTC] -> Mux3/7
  [F_PEE] -> Mux/2  "F_PEE"
  [q] -> Mux1/1
  [F_isom] -> Mux1/2
  [F_PEE] -> Mux1/3
  [B_rel] -> Mux1/4
  [F_SEE] -> Mux2/2
  [dot_l_MTC] -> Mux2/5
  [F_PEE] -> Mux2/6
  [q] -> Mux3/1
  [F_isom] -> Mux3/2
  [F_PEE] -> Mux3/3
  [F_SEE] -> Mux3/4
  [B_rel] -> Mux3/5
  Mux4/1 -> Arel eccentric/1
  [F_isom] -> Mux4/3
  [l_CE] -> Mux4/2
  [q] -> Mux4/1
  [q] -> Mux5/1
  [F_isom] -> Mux5/2
  A_rel_con/1 -> Mux5/3
  B_rel_con/1 -> Mux5/4
  Mux5/1 -> Brel1/1

== stateflow chart Library_Muscle_implementation_Ver_01/Chart ==
  state EP1
    during:
    U1=u1_EP1
    U2=u2_EP1
  state EP2
    during:
    U1=u1_EP2
    U2=u2_EP2
  (default) -> EP1
  EP1 -> EP2 : after(time_EP1,sec)
  EP2 -> EP1 : after(time_EP2,sec)
  data: U1 output; U2 output; u1_EP1 input; u1_EP2 input; u2_EP1 input; u2_EP2 input; time_EP1 input; time_EP2 input
